simulink model "second"  (R2018b)
settings: Solver=VariableStepAuto  StartTime=0.0  StopTime=7  MaxStep=0.01  RelTol=1e-3
undefined symbols (not defined in the file): sigbuilder_block
settings Model: Creator=kekos  LastModifiedBy=kekos

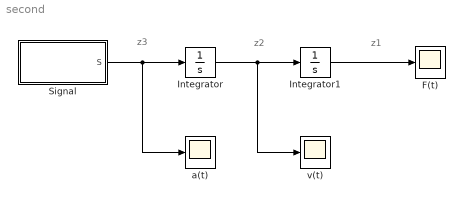
== system second ==
  note: z3
  note: z2
  note: z1
  F(t) : Scope
  Integrator : Integrator
  Integrator1 : Integrator
  Signal : Subsystem  Tag=STV Subsys  LoadFcn=sigbuilder_block('load');  StartFcn=sigbuilder_block('start');  StopFcn=sigbuilder_block('stop');  ClipboardFcn=sigbuilder_block('clipboard');  mask(Sigbuilder block){tuvar=[0:10]}
      mask help: Simulink:masks:SigbuilderBlock_MD
      mask init:
      | if ~strcmp(get_param(bdroot(gcbh),'SimulationStatus'),'stopped') tuvar = sigbuilder_block('maskInit'); end
      settings: CopyFcn=sigbuilder_block('copy');  DeleteFcn=sigbuilder_block('delete');  ModelCloseFcn=sigbuilder_block('modelClose');  PreSaveFcn=sigbuilder_block('preSave');  PauseFcn=sigbuilder_block('pause');  ContinueFcn=sigbuilder_block('continue');  NameChangeFcn=sigbuilder_block('namechange');  OpenFcn=sigbuilder_block('open',[416.4 154.2 550.8 400.2 ]);  CloseFcn=sigbuilder_block('close');
      mask Display: plot(0, 0, 100, 100,[2, 2, 32, 32, 2], [68, 8, 8, 68, 68],[32, 2], [38, 38], [32, 19, 2],[53, 60, 44], [32, 17, 17, 2],[16, 16, 31, 31]);txt = getActiveGroup(gcbh);text(2, 100, txt,'verticalAlignment', 'top');
  a(t) : Scope
  v(t) : Scope
  wires:
  Signal/1(S) -> a(t)/1, Integrator/1
  Integrator/1 -> v(t)/1, Integrator1/1
  Integrator1/1 -> F(t)/1

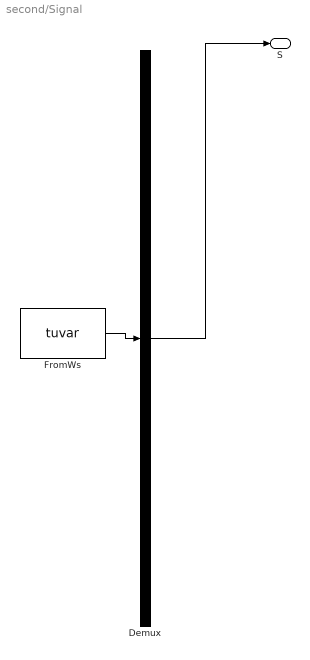
== system second/Signal ==
  Demux : Demux  Tag=STV Demux  Outputs=1
  FromWs : FromWorkspace  Tag=STV FromWs  VariableName=tuvar  SampleTime=0
      SigBuilderData=|
      | common.afterFinalStr = 'Extrapolate'
      | common.sampleTime = 0
      | dataSet.timeRange = [0 7]
      | dataSet.name = 'Group 1'
      | sbobj.Groups.Name = 'Group 1'
      | sbobj.Groups.Signals.Name = 'S'
      | sbobj.Groups.Signals.XData = [0 2 2 4.16666666667 4.16666666667 6.16666666667 6.16666666667 7]
      | sbobj.Groups.Signals.YData = [3 3 0 0 -3 -3 0 0]
      | sbobj.Groups.TimeRange = [0 7]
  S : Outport  Tag=STV Outport
  wires:
  Demux/1 -> S/1
  FromWs/1 -> Demux/1
